simulink model "motorHarness"  (R2025b)
settings: Solver=VariableStepAuto  StartTime=0.0  StopTime=80  RelTol=1e-3
libraries: eeGeneralControl x1
settings Model: Creator=karadeli  LastModifiedBy=karadeli

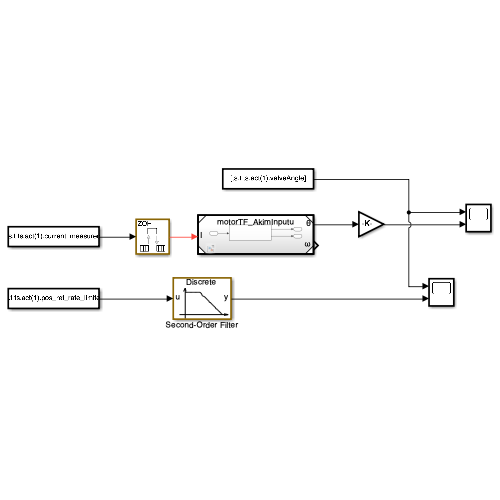
[thumbnail: Simulink's stored preview of the top-level diagram]
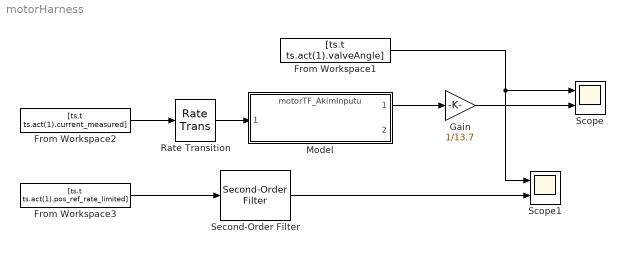
== system motorHarness ==
  From Workspace1 : FromWorkspace  VariableName=[ts.t ts.act(1).valveAngle]
  From Workspace2 : FromWorkspace  VariableName=[ts.t ts.act(1).current_measured]
  From Workspace3 : FromWorkspace  VariableName=[ts.t ts.act(1).pos_ref_rate_limited]
  Gain : Gain  Gain=1/13.7
  Model : ModelReference  ModelNameDialog=motorTF_AkimInputu.slx  SimulationMode=Normal  ModelReferenceVersion=1.10
  Rate Transition : RateTransition  OutPortSampleTime=1/8000
  Scope : Scope  NumInputPorts=2
      settings: ActiveDisplayYMinimum=-1228.0750059916045  ActiveDisplayYMaximum=7741.7734715918914
  Scope1 : Scope  NumInputPorts=2
      settings: ActiveDisplayYMinimum=-98.982884350070208  ActiveDisplayYMaximum=1098.0286485216957
  Second-Order Filter : eeGeneralControl/Second-Order Filter  FilterType=Low-pass  fn=20  Zeta=0.8  Ts=-1  A0=0  Ph0=0  f0=0  b0=0
      settings: LibrarySourceBlock=ee_sl_lib/General Control/Second-Order Filter
  wires:
  From Workspace2/1 -> Rate Transition/1
  From Workspace1/1 -> Scope1/1, Scope/1
  Model/1 -> Gain/1
  Rate Transition/1 -> Model/1
  Gain/1 -> Scope/2
  From Workspace3/1 -> Second-Order Filter/1
  Second-Order Filter/1 -> Scope1/2
